simulink model "QPSK_send_new"  (Simulink 9.0)
settings: Solver=FixedStepDiscrete  StartTime=0.0  StopTime=L*1e-4*2  RelTol=1e-3
PreLoadFcn:
  | setenv('MW_MINGW64_LOC','C:\TDM-GCC-64')
  | load('qpsktxrx.mat')
StartFcn:
  | load('qpsktxrx.mat')
  | tic
StopFcn:
  | toc;
values from neighbouring files (symbols this model uses):
  data_send = [data_send frame]    [myimg_transfer.m]    (also in test_data.m = [data_send, head, data(i:i+20*9-1)]; test_data_v2.m = [data_send, frame])
  L = length(data_send)    [myimg_transfer.m]
  qpsktxrx =     [qpsktxrx.mat]
undefined symbols (not defined in the file or in its folder): CRC, gcbh, rcfiltgaincompat
libraries: UN_HIL_Lib x2, commcrc2 x1, commutil2 x1, dspsigops x1, commsequence2 x1, commdigbbndpm3 x1, commfilt2 x1
Description:
  | QPSK Transmitter and Receiver.
  | 
  | This model shows the implementation of a QPSK transmitter and receiver.
settings Model: FPTRunName=Active  Creator=The MathWorks Inc.  LastModifiedBy=Administrator
settings DataIOCC: LimitDataPoints=on  SignalLoggingSaveFormat=ModelDataLogs  SaveOutput=off  SaveTime=off
settings OptimizationCC: BooleanDataType=off  DefaultParameterBehavior=Inlined  ExpressionDepthLimit=2147483647  LocalBlockOutputs=off
settings DebuggingCC: AlgebraicLoopMsg=error  SolverPrmCheckMsg=warning  SingleTaskRateTransMsg=error  ParameterPrecisionLossMsg=none  FcnCallInpInsideContextMsg=warning  StateNameClashWarn=warning
settings HardwareCC: TargetBitPerPointer=64  TargetBitPerSizeT=64  TargetBitPerPtrDiffT=64  TargetLongLongMode=on  TargetIntDivRoundTo=Zero  TargetEndianess=LittleEndian  TargetWordSize=64  TargetHWDeviceType=Generic->MATLAB Host Computer  ProdEqTarget=off
settings GRTTargetCC: GeneratePreprocessorConditionals=Disable all
settings ConfigComp: CovSFcnEnable=off
settings SimEventsCC: propDiagStatOutput=1  propPreventDuplicateEvents=0

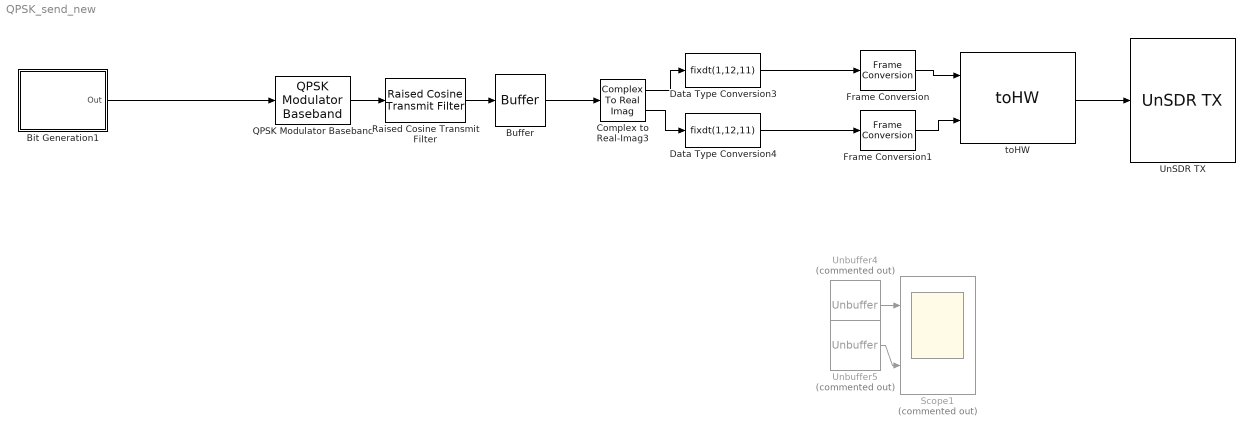
== system QPSK_send_new ==
  Bit Generation1 : Subsystem
      mask Display: disp('Bits Generation')
  Buffer : Buffer  N=4096  OutputFrames=off
  Complex to Real-Imag3 : ComplexToRealImag
  Data Type Conversion3 : DataTypeConversion  OutDataTypeStr=fixdt(1,12,11)
  Data Type Conversion4 : DataTypeConversion  OutDataTypeStr=fixdt(1,12,11)
  Frame Conversion : FrameConversion  InheritSamplingMode=off  OutFrame=Sample-based
  Frame Conversion1 : FrameConversion  InheritSamplingMode=off  OutFrame=Sample-based
  QPSK Modulator Baseband : commdigbbndpm3/QPSK Modulator Baseband  InType=Bit  Enc=Gray  Ph=pi/4  outDtype=double  outWordLen=16  outUDDataType=sfix(16)  outFracLenMode=Best precision  outFracLen=15  outDataTypeStr=double  outLastDataTypeStr=double
  Raised Cosine Transmit Filter : commfilt2/Raised Cosine Transmit Filter  filtType=Square root  R=0.5  filtSpan=2*((qpsktxrx.RaisedCosineFilterSpan)/2)  N=qpsktxrx.Upsampling  filterGain=rcfiltgaincompat(gcbh)  InputProcessing=Columns as channels (frame based)  RateOptions=Enforce single-rate processing  framing=Mute  checkCoeff=off  variableName=rcTxFilt  checkGain=Normalized  sampMode=Mute  saveAsFlag=0  currentFiltSpan=2*((qpsktxrx.RaisedCosineFilterSpan)/2)  D=(qpsktxrx.RaisedCosineFilterSpan)/2  launchFVT=off  roundingMode=Floor  overflowMode=off  coeffDataTypeStr=Inherit: Same word length as input  coeffMin=[]  coeffMax=[]  coeffLastDataTypeStr=Inherit: Same word length as input  outputDataTypeStr=Inherit: Same as accumulator  outputMin=[]  outputMax=[]  outputLastDataTypeStr=Inherit: Same as accumulator
  Scope1 : Scope  Commented=on  NumInputPorts=2
  UnSDR TX : UN_HIL_Lib/UnSDR TX  SystemSampleTime=-1
      settings: SourceProductName=HIL Blockset
  Unbuffer4 : Unbuffer  Commented=on
  Unbuffer5 : Unbuffer  Commented=on
  toHW : UN_HIL_Lib/toHW  SystemSampleTime=-1
      settings: SourceProductName=HIL Blockset
  wires:
  Unbuffer5/1 -> Scope1/2
  Unbuffer4/1 -> Scope1/1
  Data Type Conversion3/1 -> Frame Conversion/1
  Data Type Conversion4/1 -> Frame Conversion1/1
  Complex to Real-Imag3/2 -> Data Type Conversion4/1
  Complex to Real-Imag3/1 -> Data Type Conversion3/1
  QPSK Modulator Baseband/1 -> Raised Cosine Transmit Filter/1
  toHW/1 -> UnSDR TX/1
  Frame Conversion/1 -> toHW/1
  Frame Conversion1/1 -> toHW/2
  Raised Cosine Transmit Filter/1 -> Buffer/1
  Buffer/1 -> Complex to Real-Imag3/1
  Bit Generation1/1(Out) -> QPSK Modulator Baseband/1

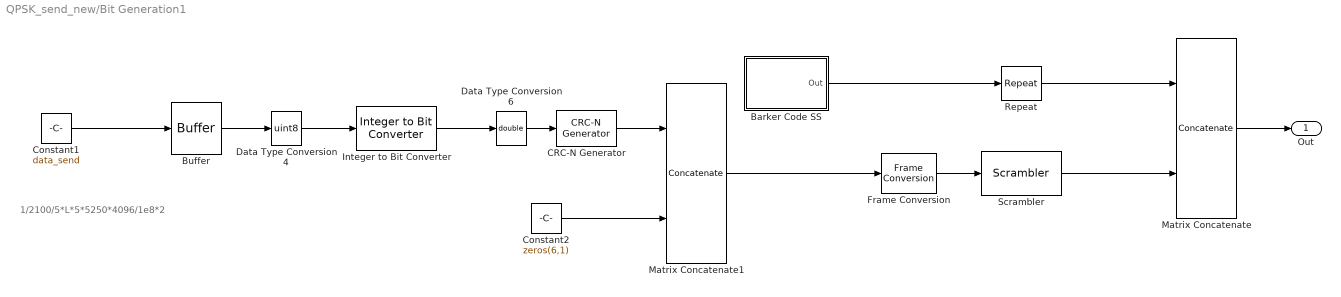
== system QPSK_send_new/Bit Generation1 ==
  note: 1/2100/5*L*5*5250*4096/1e8*2
  Barker Code SS : Subsystem
      mask Display: disp('Unipolar\nBarker Code')
  Buffer : Buffer  N=20  OutputFrames=off
  CRC-N Generator : commcrc2/CRC-N Generator  crcMethod=CRC-8  iniStates=[0]  numChecksums=1
      settings: SourceProductName=Communications System Toolbox  SourceProductBaseCode=CM
  Constant1 : Constant  Value=data_send  SampleTime=L*1e-4
  Constant2 : Constant  Value=zeros(6,1)  VectorParams1D=off  SampleTime=-1
  Data Type Conversion4 : DataTypeConversion  OutDataTypeStr=uint8
  Data Type Conversion6 : DataTypeConversion  OutDataTypeStr=double
  Frame Conversion : FrameConversion  InheritSamplingMode=off  OutFrame=Sample-based
  Integer to Bit Converter : commutil2/Integer to Bit Converter  nbits=8  signedInputValues=Unsigned  bitOrder=MSB first  outDtype=Inherit via internal rule
  Matrix Concatenate : Concatenate  Mode=Multidimensional array
  Matrix Concatenate1 : Concatenate  Mode=Multidimensional array
  Repeat : dspsigops/Repeat  N=2  InputProcessing=Columns as channels (frame based)  RateOptions=Enforce single-rate processing  ic=0  mode=Unused parameter value
      settings: SourceProductName=DSP System Toolbox
  Scrambler : commsequence2/Scrambler  M=2  poly=[1 1 1 0 1]  iniStaSource=Dialog Parameter  ini_sta=[0 0 0 0]  resetViaPort=off
      settings: SourceProductName=Communications System Toolbox  SourceProductBaseCode=CM
  Out : Outport
  wires:
  Constant2/1 -> Matrix Concatenate1/2
  Buffer/1 -> Data Type Conversion4/1
  Frame Conversion/1 -> Scrambler/1
  Scrambler/1 -> Matrix Concatenate/2
  Repeat/1 -> Matrix Concatenate/1
  Matrix Concatenate1/1 -> Frame Conversion/1
  Matrix Concatenate/1 -> Out/1
  Barker Code SS/1(Out) -> Repeat/1
  Constant1/1 -> Buffer/1
  Integer to Bit Converter/1 -> Data Type Conversion6/1
  Data Type Conversion4/1 -> Integer to Bit Converter/1
  Data Type Conversion6/1 -> CRC-N Generator/1
  CRC-N Generator/1 -> Matrix Concatenate1/1

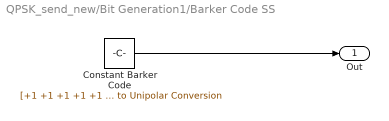
== system QPSK_send_new/Bit Generation1/Barker Code SS ==
  Constant Barker Code : Constant  Value=|  VectorParams1D=off  OutDataTypeStr=double  SampleTime=-1
      | [+1 +1 +1 +1 +1 -1 -1 +1 +1 -1 +1 -1 +1
      | ].' > 0  % Bipolar to Unipolar Conversion
  Out : Outport
  wires:
  Constant Barker Code/1 -> Out/1
